simulink model "Tilakone"  (R2020b)
settings: Solver=VariableStepAuto  StartTime=0.0  StopTime=50  RelTol=1e-3
libraries: simulink x1
settings Model: Creator=Dollar  LastModifiedBy=Dollar

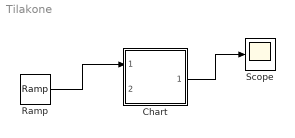
== system Tilakone ==
  Chart : Stateflow chart  TreatAsAtomicUnit=on
  Ramp : simulink/Sources/Ramp  slope=1  start=0  InitialOutput=0
  Scope : Scope
  wires:
  Chart/1(ControlSignal) -> Scope/1
  Ramp/1 -> Chart/1(Joystick)

== stateflow chart Tilakone/Chart ==
  state Control [parallel]
    settings: executionOrder=1
    state JoystickControl
      during: JoystickControl1
    state ButtonControl
    (default) -> JoystickControl
    ButtonControl -> JoystickControl : [in(Mode.JoystickMode)&&Joystick <30]
    JoystickControl -> ButtonControl : [in(Mode.ButtonMode)]
  state Mode [parallel]
    settings: executionOrder=2
    state JoystickMode
    state ButtonMode
    (default) -> JoystickMode
    ButtonMode -> JoystickMode : after(5,sec)
    JoystickMode -> ButtonMode : after(10,sec)
  data: Joystick input double; button input double; ControlSignal output double
  function JoystickControl1:
    | function JoystickControl1
    | if Joystick < 10
    |     ControlSignal = Joystick
    | else
    |     ControlSignal = 10 + (Joystick-10) * 0.1
    | end
